simulink model "planeBlock"  (R2025b)
settings: Solver=VariableStepAuto  StartTime=0.0  StopTime=80  RelTol=1e-3
model workspace (MAT data in the model file):
  Mass = 5
undefined symbols (not defined in the file): East, North, Up
libraries: simulink x2, uavutilslib x1
settings Model: Creator=Fabian  LastModifiedBy=Fabian

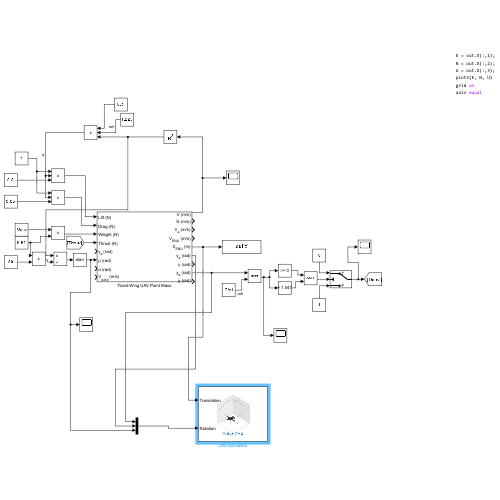
[thumbnail: Simulink's stored preview of the top-level diagram]
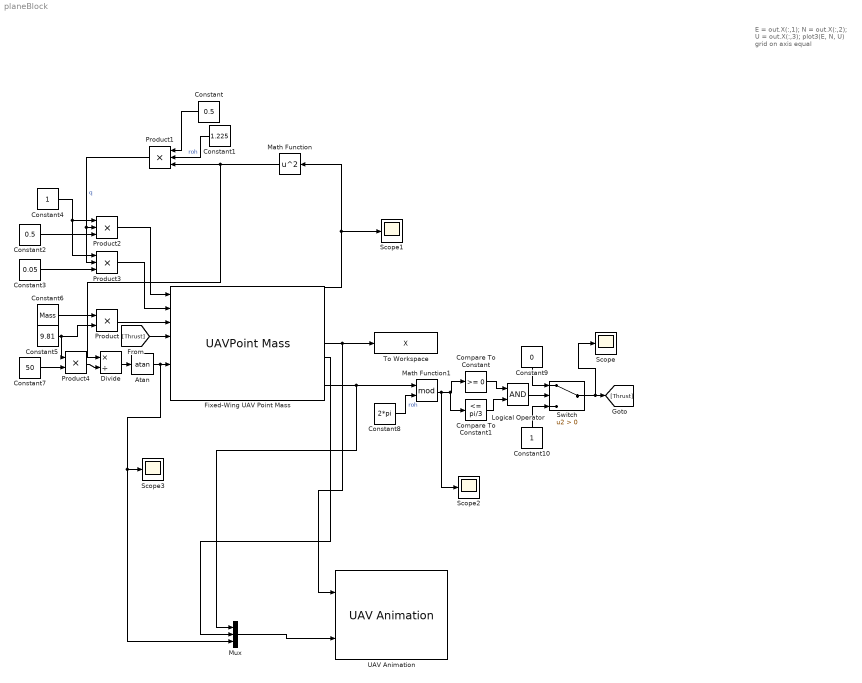
== system planeBlock ==
  note: E = out.X(:,1);
      | N = out.X(:,2);
      | U = out.X(:,3);
      | plot3(E, N, U)
      | grid on
      | axis equal
  Atan : Trigonometry  Operator=atan
  Compare To Constant : simulink/Logic and Bit Operations/Compare To Constant  relop=>=  const=0  OutDataTypeStr=boolean
  Compare To Constant1 : simulink/Logic and Bit Operations/Compare To Constant  relop=<=  const=pi/3  OutDataTypeStr=boolean
  Constant : Constant  Value=0.5
  Constant1 : Constant  Value=1.225
  Constant10 : Constant
  Constant2 : Constant  Value=0.5
  Constant3 : Constant  Value=0.05
  Constant4 : Constant
  Constant5 : Constant  Value=9.81
  Constant6 : Constant  Value=Mass
  Constant7 : Constant  Value=50
  Constant8 : Constant  Value=2*pi
  Constant9 : Constant  Value=0
  Divide : Product  Inputs=*/
  Fixed-Wing UAV Point Mass : UAVPointMass  frame=[East North Up]  altitude=100  mass=Mass
  Logical Operator : Logic  AllPortsSameDT=off  OutDataTypeStr=boolean
  Math Function : Math  Operator=square
  Math Function1 : Math  Operator=mod
  Mux : Mux  Inputs=3
  Product : Product
  Product1 : Product  Inputs=3
  Product2 : Product  Inputs=3
  Product3 : Product  Inputs=3
  Product4 : Product
  Scope{,1..3} (4 alike) : Scope
      Scope settings: ActiveDisplayYMinimum=-8.8832634386459887E+8  ActiveDisplayYMaximum=1.0977500486129756E+9
      Scope1 settings: ActiveDisplayYMinimum=-15.565305328587904  ActiveDisplayYMaximum=68.043044496206022
      Scope2 settings: ActiveDisplayYMinimum=-1626.8650415514041  ActiveDisplayYMaximum=2936.8855764201  DataLoggingVariableName=ScopeData2
      Scope3 settings: ActiveDisplayYMinimum=0.029956941929669231  ActiveDisplayYMaximum=0.032623458713814134  DataLoggingVariableName=ScopeData3
  Switch : Switch  Criteria=u2 > Threshold  SaturateOnIntegerOverflow=off  InputSameDT=off
  To Workspace : ToWorkspace  VariableName=X  SampleTime=-1
  UAV Animation : uavutilslib/UAV Animation  NumUAV=1  DynamicUAVConfig=off  UAVType=FixedWing  UAVSize=1  UAVColor=[1 0 0]  UAVTrajectoryAlpha=1  InertialZDirection=Up  RotationFormat=Euler ZYX  DrawMarkers=off  SampleTime=-1
  wires:
  Fixed-Wing UAV Point Mass/1 -> Scope1/1, Math Function/1
  Product/1 -> Fixed-Wing UAV Point Mass/3
  Math Function/1 -> Divide/1, Product1/3
  Constant1/1 -> Product1/2  "roh"
  Constant/1 -> Product1/1
  Product3/1 -> Fixed-Wing UAV Point Mass/2
  Product2/1 -> Fixed-Wing UAV Point Mass/1
  Constant3/1 -> Product3/3
  Constant2/1 -> Product2/3
  Product1/1 -> Product3/2, Product2/2  "q"
  Constant4/1 -> Product3/1, Product2/1
  Constant5/1 -> Product4/1, Product/2
  Constant6/1 -> Product/1
  Fixed-Wing UAV Point Mass/5 -> UAV Animation/1, To Workspace/1
  Constant7/1 -> Product4/2
  Atan/1 -> Mux/3, Scope3/1, Fixed-Wing UAV Point Mass/6
  Divide/1 -> Atan/1
  Product4/1 -> Divide/2
  Constant8/1 -> Math Function1/2  "roh"
  Math Function1/1 -> Scope2/1, Compare To Constant1/1, Compare To Constant/1
  Compare To Constant1/1 -> Logical Operator/2
  Compare To Constant/1 -> Logical Operator/1
  Logical Operator/1 -> Switch/2
  Constant9/1 -> Switch/1
  Constant10/1 -> Switch/3
  Switch/1 -> Scope/1, [Thrust]
  [Thrust] -> Fixed-Wing UAV Point Mass/4
  Fixed-Wing UAV Point Mass/8 -> Mux/1, Math Function1/1
  Fixed-Wing UAV Point Mass/6 -> Mux/2
  Mux/1 -> UAV Animation/2
